simulink model "simulink_lqr"  (R2023a)
settings: Solver=VariableStepAuto  StartTime=0.0  StopTime=5  RelTol=1e-3
values from neighbouring files (symbols this model uses):
  KK = lqr(A,B,Q,R)    [LQR_controller.m]
undefined symbols (not defined in the file or in its folder): aa, Asim, bb, Bsim, cc, Csim, dd, Dsim, ee, ff, mm, nn, oo, thetastart, thetastartdelta, xstart, xstartdelta
settings Model: Creator=Wolfgang  LastModifiedBy=Wolfgang
settings OptimizationCC: ReuseModelBlockBuffer=off

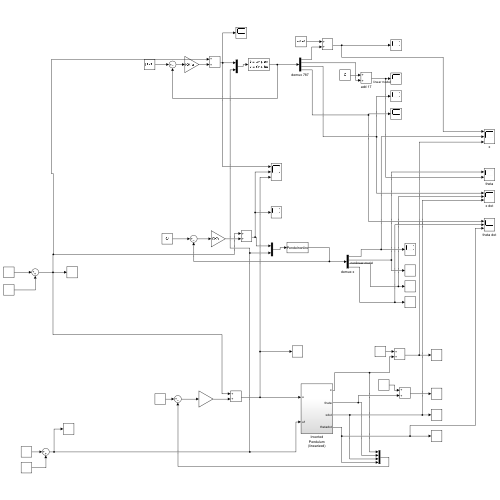
[thumbnail: Simulink's stored preview of the top-level diagram]
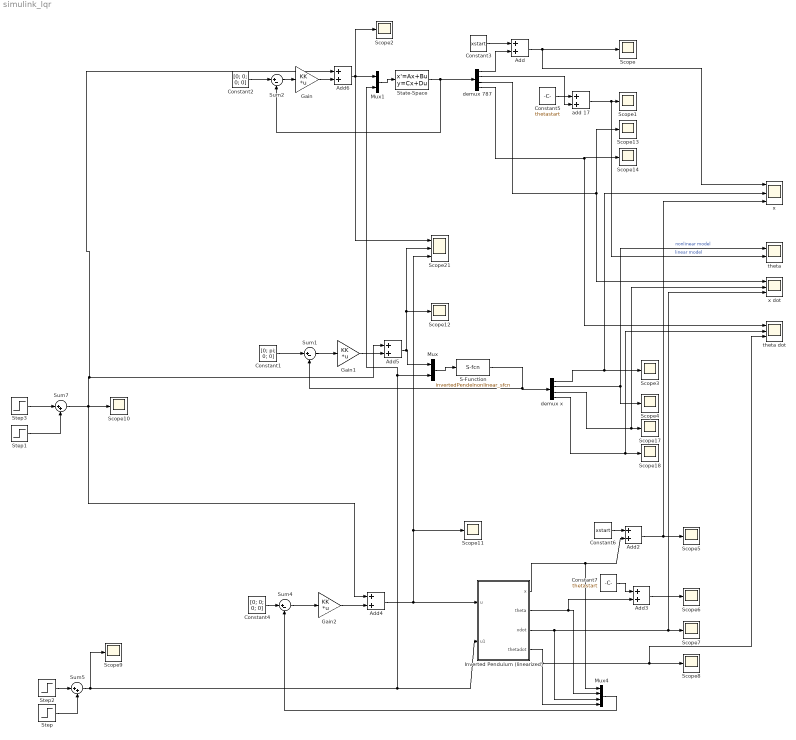
== system simulink_lqr ==
  Add{,2..6} (6 alike) : Sum
  Constant1 : Constant  Value=[0; pi; 0; 0]
  Constant2 : Constant  Value=[0; 0; 0; 0]
  Constant3 : Constant  Value=xstart
  Constant4 : Constant  Value=[0; 0; 0; 0]
  Constant5 : Constant  Value=thetastart
  Constant6 : Constant  Value=xstart
  Constant7 : Constant  Value=thetastart
  Gain : Gain  Gain=KK  Multiplication=Matrix(K*u)
  Gain1 : Gain  Gain=KK  Multiplication=Matrix(K*u)
  Gain2 : Gain  Gain=KK  Multiplication=Matrix(K*u)
  Inverted Pendulum (linearized) : Subsystem
  Mux : Mux  Inputs=2
  Mux1 : Mux  Inputs=2
  Mux4 : Mux
  S-Function : S-Function  FunctionName=invertedPendelnonlinear_sfcn  Parameters=xstart+xstartdelta; thetastart+thetastartdelta; 0; 0  SFunctionDeploymentMode=off  EnableBusSupport=off
  Scope{,1..14,17..18} (17 alike) : Scope
  Scope21 : Scope  NumInputPorts=3
  State-Space : StateSpace  A=Asim  B=Bsim  C=Csim  D=Dsim  InitialCondition=[xstartdelta; thetastartdelta; 0;0]
  Step : Step  Time=8.1  After=0  SampleTime=0
  Step1 : Step  Time=5.1  After=0  SampleTime=0
  Step2 : Step  Time=8  After=0  SampleTime=0
  Step3 : Step  Time=5  After=0  SampleTime=0
  Sum1 : Sum  Inputs=|+-
  Sum2 : Sum  Inputs=|+-
  Sum4 : Sum  Inputs=|+-
  Sum5 : Sum  Inputs=|++
  Sum7 : Sum  Inputs=|++
  add 17 : Sum
  demux 787 : Demux
  demux x : Demux
  theta : Scope  NumInputPorts=2
  theta dot : Scope  NumInputPorts=3
  x : Scope  NumInputPorts=3
  x dot : Scope  NumInputPorts=3
  wires:
  Gain/1 -> Add6/2
  State-Space/1 -> Sum2/2, demux 787/1
  Gain1/1 -> Add5/2
  Sum1/1 -> Gain1/1
  Constant1/1 -> Sum1/1
  S-Function/1 -> demux x/1, Sum1/2
  demux x/2 -> Scope4/1, theta/1  "nonlinear model"
  Constant4/1 -> Sum4/1
  Inverted Pendulum (linearized)/4(thetadot) -> Mux4/4, theta dot/3, Scope8/1
  Inverted Pendulum (linearized)/2(theta) -> Add3/2, Mux4/2
  Inverted Pendulum (linearized)/1(x) -> Add2/2, Mux4/1
  Mux4/1 -> Sum4/2
  Inverted Pendulum (linearized)/3(xdot) -> Mux4/3, x dot/3, Scope7/1
  Sum4/1 -> Gain2/1
  Sum5/1 -> Mux1/2, Mux/2, Inverted Pendulum (linearized)/2(u1), Scope9/1
  Step2/1 -> Sum5/1
  Step/1 -> Sum5/2
  Add4/1 -> Inverted Pendulum (linearized)/1(u), Scope11/1, Scope21/3
  Gain2/1 -> Add4/2
  Sum7/1 -> Add6/1, Add5/1, Add4/1, Scope10/1
  Step3/1 -> Sum7/1
  Step1/1 -> Sum7/2
  demux 787/2 -> add 17/2
  demux x/1 -> x/2, Scope3/1
  Constant2/1 -> Sum2/1
  Sum2/1 -> Gain/1
  demux 787/3 -> x dot/1, Scope13/1
  demux 787/4 -> theta dot/1, Scope14/1
  demux 787/1 -> Add/2
  Add/1 -> x/1, Scope/1
  Constant3/1 -> Add/1
  add 17/1 -> theta/2, Scope1/1  "linear model"
  Constant5/1 -> add 17/1
  demux x/3 -> x dot/2, Scope17/1
  demux x/4 -> theta dot/2, Scope18/1
  Constant6/1 -> Add2/1
  Add2/1 -> x/3, Scope5/1
  Add3/1 -> Scope6/1
  Constant7/1 -> Add3/1
  Add5/1 -> Scope21/2, Scope12/1, Mux/1
  Add6/1 -> Scope21/1, Mux1/1, Scope2/1
  Mux/1 -> S-Function/1
  Mux1/1 -> State-Space/1

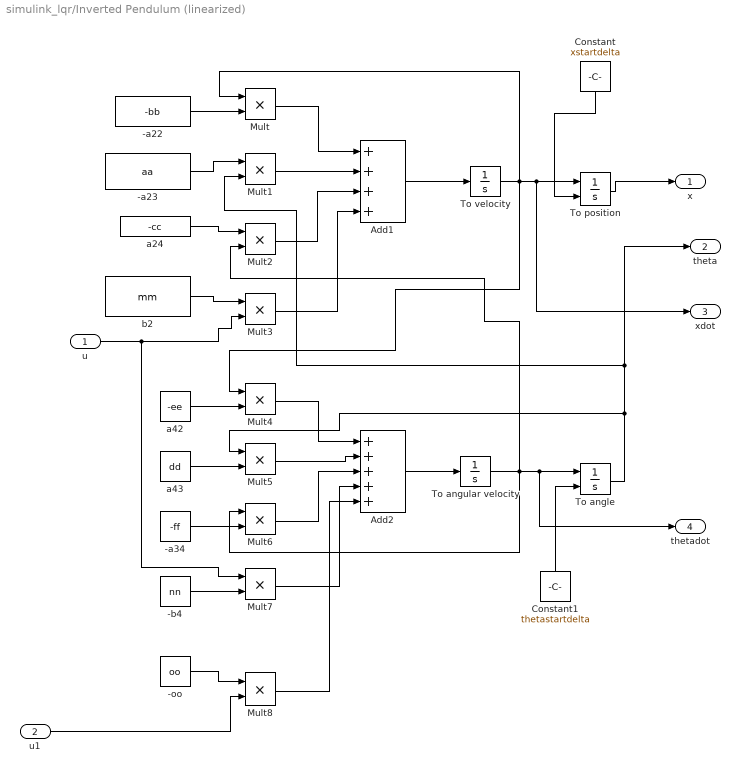
== system simulink_lqr/Inverted Pendulum (linearized) ==
  u : Inport
  u1 : Inport  Port=2
  -a22 : Constant  Value=-bb
  -a23 : Constant  Value=aa
  -a34 : Constant  Value=-ff
  -b4 : Constant  Value=nn
  -oo : Constant  Value=oo
  Add1 : Sum  Inputs=++++
  Add2 : Sum  Inputs=+++++
  Constant : Constant  Value=xstartdelta
  Constant1 : Constant  Value=thetastartdelta
  Mult{,1..8} (9 alike) : Product  Inputs=**
  To angle : Integrator  InitialConditionSource=external  InitialCondition=1.5
  To angular velocity : Integrator
  To position : Integrator  InitialConditionSource=external  InitialCondition=1
  To velocity : Integrator
  a24 : Constant  Value=-cc
  a42 : Constant  Value=-ee
  a43 : Constant  Value=dd
  b2 : Constant  Value=mm
  x : Outport  VectorParamsAs1DForOutWhenUnconnected=off
  theta : Outport  Port=2  VectorParamsAs1DForOutWhenUnconnected=off
  xdot : Outport  Port=3  VectorParamsAs1DForOutWhenUnconnected=off
  thetadot : Outport  Port=4  VectorParamsAs1DForOutWhenUnconnected=off
  wires:
  -a22/1 -> Mult/2
  Add2/1 -> To angular velocity/1
  -a34/1 -> Mult6/2
  -b4/1 -> Mult7/2
  Mult6/1 -> Add2/3
  Mult3/1 -> Add1/4
  Mult1/1 -> Add1/2
  Add1/1 -> To velocity/1
  b2/1 -> Mult3/1
  To angular velocity/1 -> Mult6/1, Mult2/2, thetadot/1, To angle/1
  -a23/1 -> Mult1/1
  To velocity/1 -> Mult4/1, Mult/1, xdot/1, To position/1
  To angle/1 -> theta/1, Mult1/2, Mult5/1
  Mult7/1 -> Add2/4
  a43/1 -> Mult5/2
  Mult4/1 -> Add2/1
  Mult2/1 -> Add1/3
  u/1 -> Mult7/1, Mult3/2
  a42/1 -> Mult4/2
  Mult/1 -> Add1/1
  Mult5/1 -> Add2/2
  a24/1 -> Mult2/1
  To position/1 -> x/1
  Constant1/1 -> To angle/2
  Constant/1 -> To position/2
  Mult8/1 -> Add2/5
  -oo/1 -> Mult8/1
  u1/1 -> Mult8/2
